simulink model "rstr_modelR2015a"  (R2015a)
settings: Solver=ode45  SolverMode=SingleTasking  StartTime=0.0  StopTime=20  RelTol=1e-3
values from neighbouring files (symbols this model uses):
  Ar = [0      1 0      0 0   0 ... (first row only)    [desafio1.m]
  Br = [0   0   0   0 ... (first row only)    [desafio1.m]
  Cr = [1 0 0 0 0 0 ... (first row only)    [desafio1.m]
  Fr = -lqr(Ar,Br,eye(6),eye(4),0)    [desafio1.m]
  Kr = lqr(Ar.',Cr.',eye(6),eye(2),0)'    [desafio1.m]
  r = [1; 5]    [desafio1.m]
  sim_step = 0.001    [desafio1.m]
  x0r = [x0; 0; 0]    [desafio1.m]
libraries: simulink x1
settings Model: CovMetricSettings=dwe  CovHtmlReporting=off  covSaveCumulativeToWorkspaceVar=off  CovSaveSingleToWorkspaceVar=off  CovExternalEMLEnable=on  Creator=vinic  LastModifiedBy=vinic
settings DataIOCC: LimitDataPoints=off  SaveFormat=Dataset  ReturnWorkspaceOutputs=on
settings DebuggingCC: SFUnexpectedBacktrackingDiag=error  SFNoUnconditionalDefaultTransitionDiag=error
settings HardwareCC: ProdBitPerPointer=64  ProdLargestAtomicFloat=Float  ProdIntDivRoundTo=Zero  ProdEndianess=LittleEndian  ProdHWDeviceType=Specified
settings ModelReferenceCC: PropagateSignalLabelsOutOfModel=on
settings SFSimCC: SimUseLocalCustomCode=on
settings RTWCC: RTWUseLocalCustomCode=on
settings GRTTargetCC: TargetLangStandard=C99 (ISO)

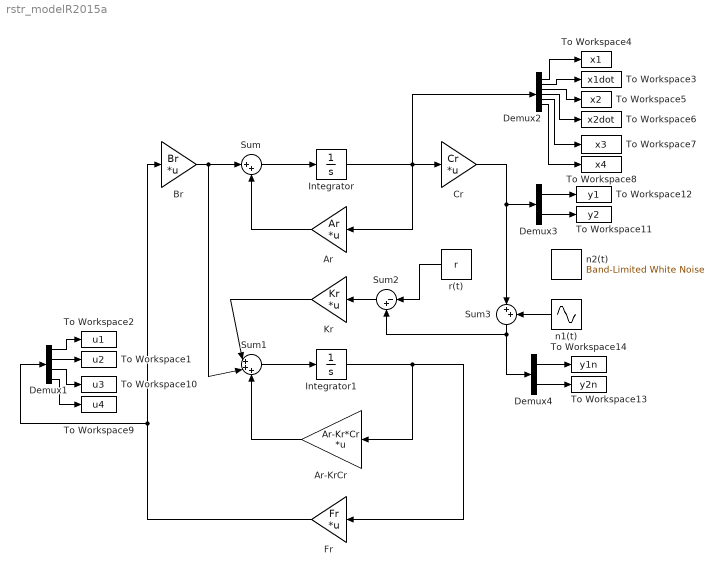
== system rstr_modelR2015a ==
  Ar : Gain  Gain=Ar  Multiplication=Matrix(K*u)
  Ar-KrCr : Gain  Gain=Ar-Kr*Cr  Multiplication=Matrix(K*u)
  Br : Gain  Gain=Br  Multiplication=Matrix(K*u)
  Cr : Gain  Gain=Cr  Multiplication=Matrix(K*u)
  Demux1 : Demux
  Demux2 : Demux  Outputs=6
  Demux3 : Demux  Outputs=2
  Demux4 : Demux  Outputs=2
  Fr : Gain  Gain=Fr  Multiplication=Matrix(K*u)
  Integrator : Integrator  InitialCondition=x0r
  Integrator1 : Integrator
  Kr : Gain  Gain=Kr  Multiplication=Matrix(K*u)
  Sum : Sum  Inputs=|++
  Sum1 : Sum  Inputs=|+++
  Sum2 : Sum  Inputs=|-+
  Sum3 : Sum  Inputs=|++
  To Workspace1 : ToWorkspace  VariableName=u2  SampleTime=-1
      settings: Save2DSignal=2-D array (concatenate along first dimension)
  To Workspace10 : ToWorkspace  VariableName=u3  SampleTime=-1
      settings: Save2DSignal=2-D array (concatenate along first dimension)
  To Workspace11 : ToWorkspace  VariableName=y2  SampleTime=-1
      settings: Save2DSignal=2-D array (concatenate along first dimension)
  To Workspace12 : ToWorkspace  VariableName=y1  SampleTime=-1
      settings: Save2DSignal=2-D array (concatenate along first dimension)
  To Workspace13 : ToWorkspace  VariableName=y2n  SampleTime=-1
      settings: Save2DSignal=2-D array (concatenate along first dimension)
  To Workspace14 : ToWorkspace  VariableName=y1n  SampleTime=-1
      settings: Save2DSignal=2-D array (concatenate along first dimension)
  To Workspace2 : ToWorkspace  VariableName=u1  SampleTime=-1
      settings: Save2DSignal=2-D array (concatenate along first dimension)
  To Workspace3 : ToWorkspace  VariableName=x1dot  SampleTime=-1
      settings: Save2DSignal=2-D array (concatenate along first dimension)
  To Workspace4 : ToWorkspace  VariableName=x1  SampleTime=-1
      settings: Save2DSignal=2-D array (concatenate along first dimension)
  To Workspace5 : ToWorkspace  VariableName=x2  SampleTime=-1
      settings: Save2DSignal=2-D array (concatenate along first dimension)
  To Workspace6 : ToWorkspace  VariableName=x2dot  SampleTime=-1
      settings: Save2DSignal=2-D array (concatenate along first dimension)
  To Workspace7 : ToWorkspace  VariableName=x3  SampleTime=-1
      settings: Save2DSignal=2-D array (concatenate along first dimension)
  To Workspace8 : ToWorkspace  VariableName=x4  SampleTime=-1
      settings: Save2DSignal=2-D array (concatenate along first dimension)
  To Workspace9 : ToWorkspace  VariableName=u4  SampleTime=-1
      settings: Save2DSignal=2-D array (concatenate along first dimension)
  n1(t) : Sin  Amplitude=0.01  Frequency=100  SampleTime=0
  n2(t) : simulink/Sources/Band-Limited White Noise  Cov=[1e-4]  Ts=sim_step  seed=[23341]
  r(t) : Constant  Value=r  VectorParams1D=off
  wires:
  Kr/1 -> Sum1/1
  Demux2/1 -> To Workspace4/1
  Demux2/2 -> To Workspace3/1
  Demux1/2 -> To Workspace1/1
  Integrator1/1 -> Ar-KrCr/1, Fr/1
  Demux2/3 -> To Workspace5/1
  Demux1/1 -> To Workspace2/1
  Fr/1 -> Br/1, Demux1/1
  Ar/1 -> Sum/2
  Integrator/1 -> Ar/1, Demux2/1, Cr/1
  Ar-KrCr/1 -> Sum1/3
  Br/1 -> Sum/1, Sum1/2
  Demux2/4 -> To Workspace6/1
  Sum1/1 -> Integrator1/1
  Sum/1 -> Integrator/1
  Demux2/5 -> To Workspace7/1
  Demux2/6 -> To Workspace8/1
  Demux1/3 -> To Workspace10/1
  Demux1/4 -> To Workspace9/1
  Demux3/1 -> To Workspace12/1
  Demux3/2 -> To Workspace11/1
  Sum3/1 -> Sum2/2, Demux4/1
  Demux4/1 -> To Workspace14/1
  Demux4/2 -> To Workspace13/1
  Cr/1 -> Sum3/1, Demux3/1
  Sum2/1 -> Kr/1
  r(t)/1 -> Sum2/1
  n1(t)/1 -> Sum3/2
